simulink subsystem "BMSSoCDirect"  (R2024b)
settings: Solver=VariableStepAuto  StartTime=0.0  StopTime=10.0  RelTol=1e-3
settings Model: Creator=jjha  LastModifiedBy=jjha
settings OptimizationCC: ReuseModelBlockBuffer=off
settings RTWCC: GPUComputeCapability=3.5

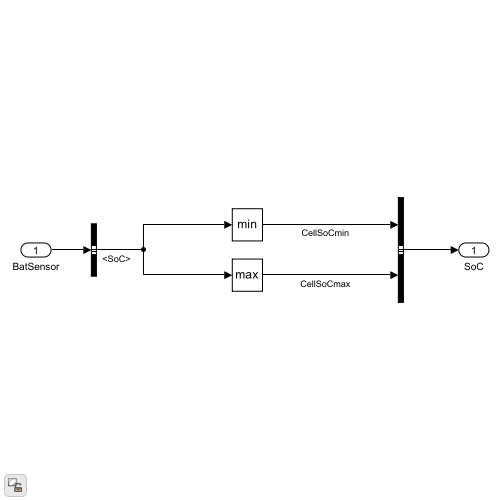
[thumbnail: Simulink's stored preview of the top-level diagram]
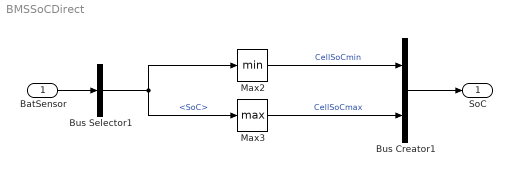
== system BMSSoCDirect ==
  BatSensor : Inport
  Bus Creator1 : BusCreator  Inputs=2
  Bus Selector1 : BusSelector  OutputSignals=SoC
  Max2 : MinMax  ZeroCross=off
  Max3 : MinMax  Function=max  ZeroCross=off
  SoC : Outport
  wires:
  BatSensor/1 -> Bus Selector1/1
  Max3/1 -> Bus Creator1/2  "CellSoCmax"
  Max2/1 -> Bus Creator1/1  "CellSoCmin"
  Bus Selector1/1 -> Max2/1, Max3/1  "<SoC>"
  Bus Creator1/1 -> SoC/1
